simulink model "lab3_simulink"  (R2023a)
settings: Solver=VariableStepAuto  StartTime=0.0  StopTime=150  RelTol=1e-3
values from neighbouring files (symbols this model uses):
  Tm = 2.5    [Laboratory3.m]
  Tm2 = 3    [Laboratory3.m]
  Ts = 0.5    [Laboratory3.m]
  Ts2 = Tm2/5    (= 0.6)    [Laboratory3.m]
undefined symbols (not defined in the file or in its folder): denF, denR, denR2, denR4, denRbun, denRe, numF, numR, numR2, numR4, numRbun, numRe
settings Model: Creator=Voic  LastModifiedBy=evely
settings OptimizationCC: ReuseModelBlockBuffer=off

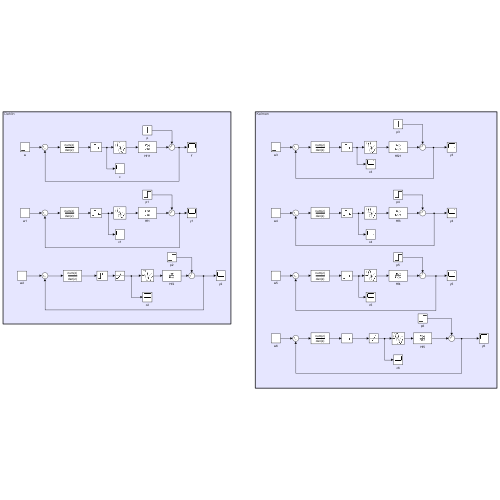
[thumbnail: Simulink's stored preview of the top-level diagram]
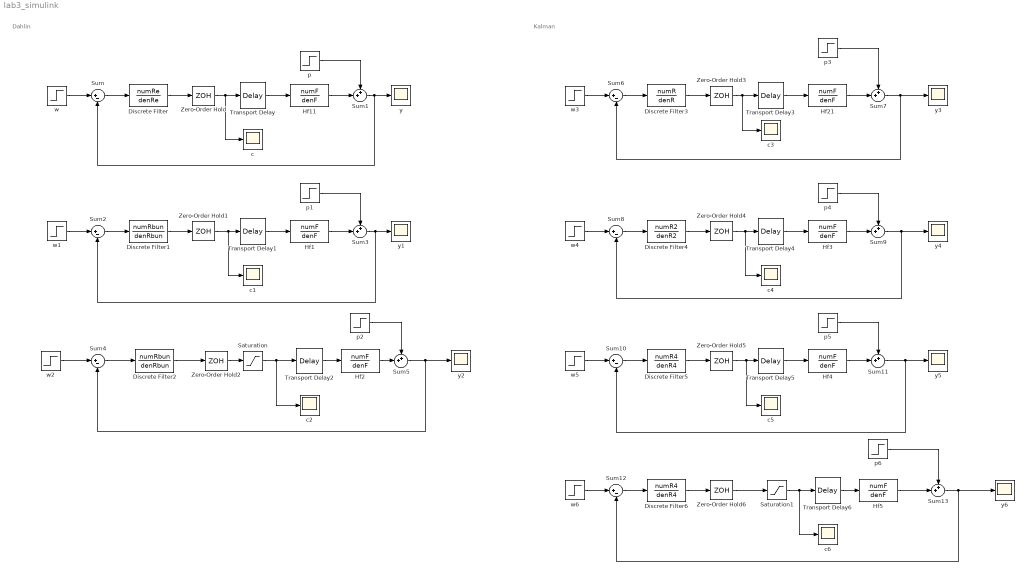
== system lab3_simulink ==
  note: Kalman
  note: Dahlin
  Discrete Filter : DiscreteFilter  Numerator=numRe  Denominator=denRe
  Discrete Filter1 : DiscreteFilter  Numerator=numRbun  Denominator=denRbun
  Discrete Filter2 : DiscreteFilter  Numerator=numRbun  Denominator=denRbun
  Discrete Filter3 : DiscreteFilter  Numerator=numR  Denominator=denR
  Discrete Filter4 : DiscreteFilter  Numerator=numR2  Denominator=denR2
  Discrete Filter5 : DiscreteFilter  Numerator=numR4  Denominator=denR4
  Discrete Filter6 : DiscreteFilter  Numerator=numR4  Denominator=denR4
  Hf{1..5,11,21} (7 alike) : TransferFcn  Numerator=numF  Denominator=denF
  Saturation : Saturate  UpperLimit=1  LowerLimit=0
  Saturation1 : Saturate  UpperLimit=1  LowerLimit=0.
  Sum{,2,4,6,8,10,12} (7 alike) : Sum  Inputs=|+-
  Sum{1,3,5,7,9,11,13} (7 alike) : Sum  Inputs=++|
  Transport Delay : TransportDelay  DelayTime=Tm
  Transport Delay1 : TransportDelay  DelayTime=Tm
  Transport Delay2 : TransportDelay  DelayTime=Tm
  Transport Delay{3..6} (4 alike) : TransportDelay  DelayTime=Tm2
  Zero-Order Hold : ZeroOrderHold  SampleTime=Ts
  Zero-Order Hold1 : ZeroOrderHold  SampleTime=Ts
  Zero-Order Hold2 : ZeroOrderHold  SampleTime=Ts
  Zero-Order Hold{3..6} (4 alike) : ZeroOrderHold  SampleTime=Ts2
  c{,1..6} (7 alike) : Scope
  p{,1..6} (7 alike) : Step  After=0  SampleTime=0
  w{,1..6} (7 alike) : Step  SampleTime=0
  y{,1..6} (7 alike) : Scope
  wires:
  p/1 -> Sum1/1
  Sum/1 -> Discrete Filter/1
  Transport Delay/1 -> Hf11/1
  Sum1/1 -> y/1, Sum/2
  Hf11/1 -> Sum1/2
  w/1 -> Sum/1
  Discrete Filter/1 -> Zero-Order Hold/1
  Zero-Order Hold/1 -> Transport Delay/1, c/1
  w1/1 -> Sum2/1
  Sum2/1 -> Discrete Filter1/1
  Sum3/1 -> y1/1, Sum2/2
  p1/1 -> Sum3/1
  Transport Delay1/1 -> Hf1/1
  Discrete Filter1/1 -> Zero-Order Hold1/1
  Hf1/1 -> Sum3/2
  Zero-Order Hold1/1 -> Transport Delay1/1, c1/1
  Zero-Order Hold2/1 -> Saturation/1
  Discrete Filter2/1 -> Zero-Order Hold2/1
  Hf2/1 -> Sum5/2
  Sum5/1 -> y2/1, Sum4/2
  w2/1 -> Sum4/1
  p2/1 -> Sum5/1
  Transport Delay2/1 -> Hf2/1
  Sum4/1 -> Discrete Filter2/1
  Saturation/1 -> Transport Delay2/1, c2/1
  Zero-Order Hold3/1 -> Transport Delay3/1, c3/1
  Hf21/1 -> Sum7/2
  Sum7/1 -> y3/1, Sum6/2
  Transport Delay3/1 -> Hf21/1
  w3/1 -> Sum6/1
  Discrete Filter3/1 -> Zero-Order Hold3/1
  Sum6/1 -> Discrete Filter3/1
  p3/1 -> Sum7/1
  Sum9/1 -> y4/1, Sum8/2
  Zero-Order Hold4/1 -> Transport Delay4/1, c4/1
  w4/1 -> Sum8/1
  Discrete Filter4/1 -> Zero-Order Hold4/1
  Sum8/1 -> Discrete Filter4/1
  Hf3/1 -> Sum9/2
  p4/1 -> Sum9/1
  Transport Delay4/1 -> Hf3/1
  Zero-Order Hold5/1 -> Transport Delay5/1, c5/1
  Sum11/1 -> y5/1, Sum10/2
  w5/1 -> Sum10/1
  Hf4/1 -> Sum11/2
  Transport Delay5/1 -> Hf4/1
  p5/1 -> Sum11/1
  Sum10/1 -> Discrete Filter5/1
  Discrete Filter5/1 -> Zero-Order Hold5/1
  Transport Delay6/1 -> Hf5/1
  Zero-Order Hold6/1 -> Saturation1/1
  p6/1 -> Sum13/1
  Discrete Filter6/1 -> Zero-Order Hold6/1
  Sum12/1 -> Discrete Filter6/1
  w6/1 -> Sum12/1
  Hf5/1 -> Sum13/2
  Sum13/1 -> y6/1, Sum12/2
  Saturation1/1 -> Transport Delay6/1, c6/1
